simulink model "WGmodel_v6"  (R2022b)
settings: Solver=VariableStepAuto  StartTime=0.0  StopTime=100  RelTol=1e-3
values from neighbouring files (symbols this model uses):
  m_pw = zeros(nvw,nwr)    [fun_getwindpowercurve_v4.m]
  pinitwindgen = 0.5161    [WGmodel_startup.m]    (also in WGmodel_startup_v2.m; WGmodel_startup_v3.m = pinitwindgen(1))
  R = 0.05    [WGmodel_startup.m]    (also in WGmodel_startup_v2.m; WGmodel_startup_v3.m)
  Tc1 = 0.05    [WGmodel_startup.m]    (also in WGmodel_startup_v2.m; WGmodel_startup_v3.m)
  Tc2 = 0.05    [WGmodel_startup.m]    (also in WGmodel_startup_v2.m; WGmodel_startup_v3.m)
  v_beta = 0:1:2    [WGmodel_startup.m]    (also in fun_getwindpowercurve_v2.m = 0.5)
  v_pwdel = 0.9 * max(m_pw,[],2)    [fun_getwindpowercurve_v2.m]    (also in fun_getwindpowercurve_v3.m = (1-deload) * v_pwmpp; fun_getwindpowercurve_v4.m = (1-deload) * v_pwmpp)
  v_vw = 5:10    [LUT_2D.m]    (also in WGmodel_startup.m = 5:1:10; WGmodel_startup_v2.m = 5:1:15; WGmodel_startup_v3.m = 5:.5:12; fun_getwindpowercurve_v2.m = [10 11 12])
  v_wr = v_Wr/Wrn    [fun_getwindpowercurve.m]    (also in fun_getwindpowercurve_v2.m; fun_getwindpowercurve_v3.m; fun_getwindpowercurve_v4.m; fun_getwindpowercurve_v5.m)
  v_wrdel = (v_wr(v_iwrmpp+i_lower)+v_wr(v_iwrmpp+i_higher))/2    [fun_getwindpowercurve_v2.m]    (also in fun_getwindpowercurve_v3.m = v_Wrdel/Wrn; fun_getwindpowercurve_v4.m = v_Wrdel/Wrn)
  wr0 = wr0(1)    [WGmodel_startup_v3.m]
settings Model: Creator=User  LastModifiedBy=User
settings DataIOCC: ReturnWorkspaceOutputsName=tp07107dd9_9efb_4f85_a9e4_60e1f7b33de8

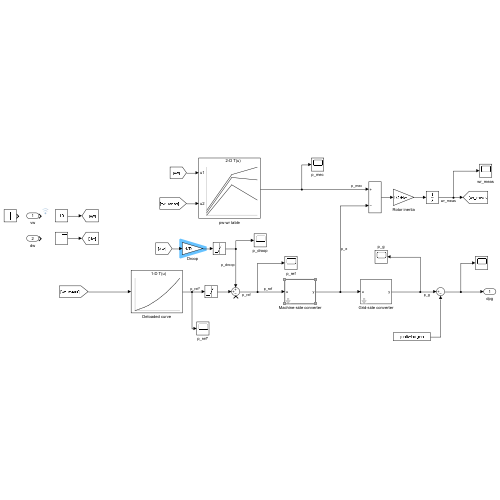
[thumbnail: Simulink's stored preview of the top-level diagram]
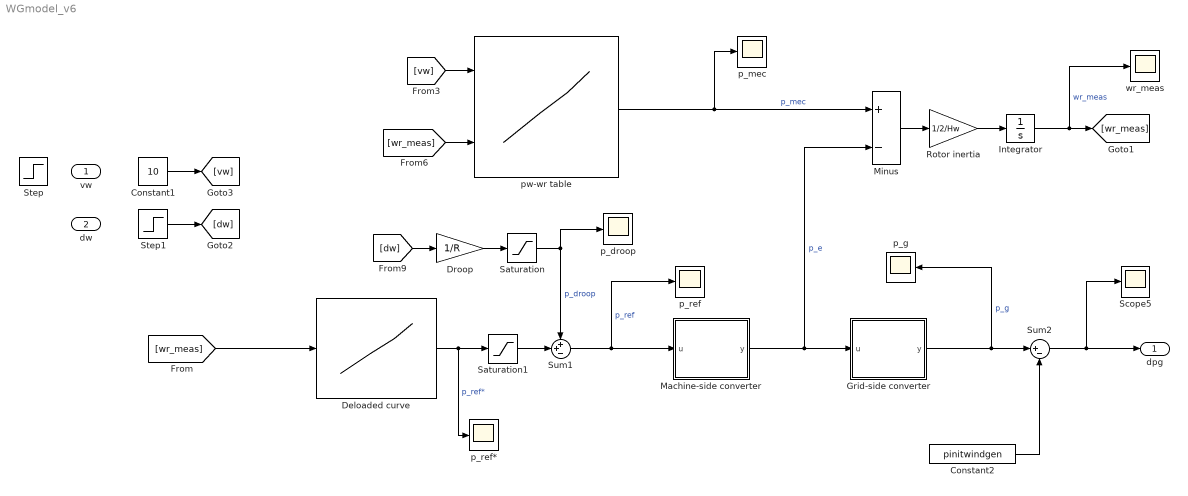
== system WGmodel_v6 ==
  vw : Inport
  dw : Inport  Port=2
  Constant1 : Constant  Value=10
  Constant2 : Constant  Value=pinitwindgen
  Deloaded curve : Lookup_n-D  NumberOfTableDimensions=1  BreakpointsForDimension1=v_wrdel  Table=v_pwdel  InternalRulePriority=Speed  RndMeth=Simplest
  Droop : Gain  Gain=1/R
  Grid-side converter : Subsystem  mask{T=Tc2, y0=pinitwindgen}
      mask prompts: T "Time constant (s)"; y0 "Initial condition (pu)"
  Integrator : Integrator  InitialCondition=wr0
  Machine-side converter : Subsystem  mask{T=Tc1, y0=pinitwindgen}
      mask prompts: T "Time constant (s)"; y0 "Initial condition (pu)"
  Minus : Sum  Inputs=+-
  Rotor inertia : Gain  Gain=1/2/Hw
  Saturation : Saturate
  Saturation1 : Saturate  UpperLimit=v_pwdel(length(v_pwdel))  LowerLimit=0
  Scope5 : Scope
  Step : Step  Time=10  Before=10  After=12  SampleTime=0
  Step1 : Step  Time=50  After=.01  SampleTime=0
  Sum1 : Sum  Inputs=++-
  Sum2 : Sum  Inputs=|+-
  p_droop : Scope
  p_g : Scope
  p_mec : Scope
  p_ref : Scope
  p_ref* : Scope
  pw-wr table : Lookup_n-D  BreakpointsForDimension1=v_vw  BreakpointsForDimension2=v_wr  BreakpointsForDimension3=v_beta  Table=m_pw  InternalRulePriority=Speed  RndMeth=Simplest
      settings: InputPortMap=u0,u1
  wr_meas : Scope
  dpg : Outport
  wires:
  Minus/1 -> Rotor inertia/1
  Integrator/1 -> wr_meas/1, [wr_meas]  "wr_meas"
  Rotor inertia/1 -> Integrator/1
  pw-wr table/1 -> Minus/1, p_mec/1  "p_mec"
  [dw] -> Droop/1
  Step1/1 -> [dw]
  Constant1/1 -> [vw]
  Constant2/1 -> Sum2/2
  Grid-side converter/1(y) -> Sum2/1, p_g/1  "p_g"
  [wr_meas] -> pw-wr table/2
  [vw] -> pw-wr table/1
  [wr_meas] -> Deloaded curve/1
  Deloaded curve/1 -> p_ref*/1, Saturation1/1  "p_ref*"
  Sum1/1 -> Machine-side converter/1(u), p_ref/1  "p_ref"
  Sum2/1 -> Scope5/1, dpg/1
  Machine-side converter/1(y) -> Minus/2, Grid-side converter/1(u)  "p_e"
  Droop/1 -> Saturation/1
  Saturation/1 -> p_droop/1, Sum1/1  "p_droop"
  Saturation1/1 -> Sum1/2

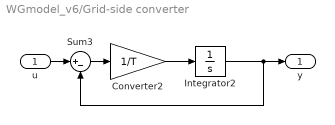
== system WGmodel_v6/Grid-side converter ==
  u : Inport
  Converter2 : Gain  Gain=1/T
  Integrator2 : Integrator  InitialCondition=y0
  Sum3 : Sum  Inputs=|+-
  y : Outport
  wires:
  Integrator2/1 -> y/1, Sum3/2
  Sum3/1 -> Converter2/1
  Converter2/1 -> Integrator2/1
  u/1 -> Sum3/1

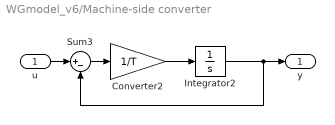
== system WGmodel_v6/Machine-side converter ==
  u : Inport
  Converter2 : Gain  Gain=1/T
  Integrator2 : Integrator  InitialCondition=y0
  Sum3 : Sum  Inputs=|+-
  y : Outport
  wires:
  Integrator2/1 -> y/1, Sum3/2
  Sum3/1 -> Converter2/1
  Converter2/1 -> Integrator2/1
  u/1 -> Sum3/1
